simulink model "ctrl"  (R2018a)
settings: Solver=FixedStepDiscrete  StartTime=0.0  StopTime=3  RelTol=1e-3  EnableMultiTasking=on
undefined symbols (not defined in the file): AutoCalSt, Cfg_EnblLoadObs, Cfg_IndIDCntThshld, Cfg_IndIDCoolDownTicks, Cfg_IndIDMaxThshld, Cfg_IndIDMinThshld, Cfg_IndIDMtrVin, Cfg_IndIDSwTicks, Cfg_IndIDTs, Cfg_ResIDCntThshld, Cfg_ResIDMaxThshld, Cfg_ResIDMinThshld, Cfg_ResIDMtrVin, Cfg_SpdSnsSrc, DiscIntNeverNeededParam, MotorParams, MtrCtrlMd
libraries: ctrl_lib x5, simulink x3, adrc_lib x2
settings Model: PauseTimes=0.1  Creator=uids8840  LastModifiedBy=elrobotista
settings SolverCC: AutoInsertRateTranBlk=on
settings DataIOCC: SaveOutput=off  SignalLogging=off  DSMLogging=off  SaveTime=off
settings OptimizationCC: DefaultParameterBehavior=Inlined  UseFloatMulNetSlope=on  InlineInvariantSignals=on  PassReuseOutputArgsAs=Individual arguments  ZeroExternalMemoryAtStartup=off  ZeroInternalMemoryAtStartup=off  NoFixptDivByZeroProtection=on  EfficientFloat2IntCast=on  LifeSpan=1
settings DebuggingCC: ParameterTunabilityLossMsg=error
settings HardwareCC: ProdBitPerPointer=32  ProdBitPerSizeT=32  ProdBitPerPtrDiffT=32  ProdLargestAtomicInteger=Long  ProdLargestAtomicFloat=Double  ProdWordSize=32  ProdHWDeviceType=ARM Compatible->ARM Cortex
settings ModelReferenceCC: ModelReferenceNumInstancesAllowed=Single
settings SFSimCC: MATLABDynamicMemAlloc=off
settings RTWCC: SystemTargetFile=ert.tlc  GenCodeOnly=on  PackageGeneratedCodeAndArtifacts=on  PackageName=mtrctl  TemplateMakefile=ert_default_tmf  GenerateReport=on  IncludeHyperlinkInReport=on  LaunchReport=on  GenerateTraceInfo=on  GenerateTraceReport=on  GenerateTraceReportSl=on  GenerateTraceReportSf=on  GenerateTraceReportEml=on  GenerateCodeMetricsReport=on
settings CodeAppCC: ForceParamTrailComments=on  IgnoreCustomStorageClasses=off  OperatorAnnotations=on  SimulinkDataObjDesc=on  SFDataObjDesc=on  CustomSymbolStrGlobalVar=rt$N$M  CustomSymbolStrType=$N$M  CustomSymbolStrFcn=$N$M$F  CustomSymbolStrMacro=$N$M  InsertBlockDesc=on
settings ERTTargetCC: TargetLangStandard=C99 (ISO)  GenerateFullHeader=off  IncludeMdlTerminateFcn=off  CombineSignalStateStructs=on  SuppressErrorStatus=on  ERTCustomFileBanners=off  SupportAbsoluteTime=off  SupportNonFinite=off  SupportComplex=off  InlinedParameterPlacement=NonHierarchical  ERTCustomFileTemplate=example_file_process.tlc

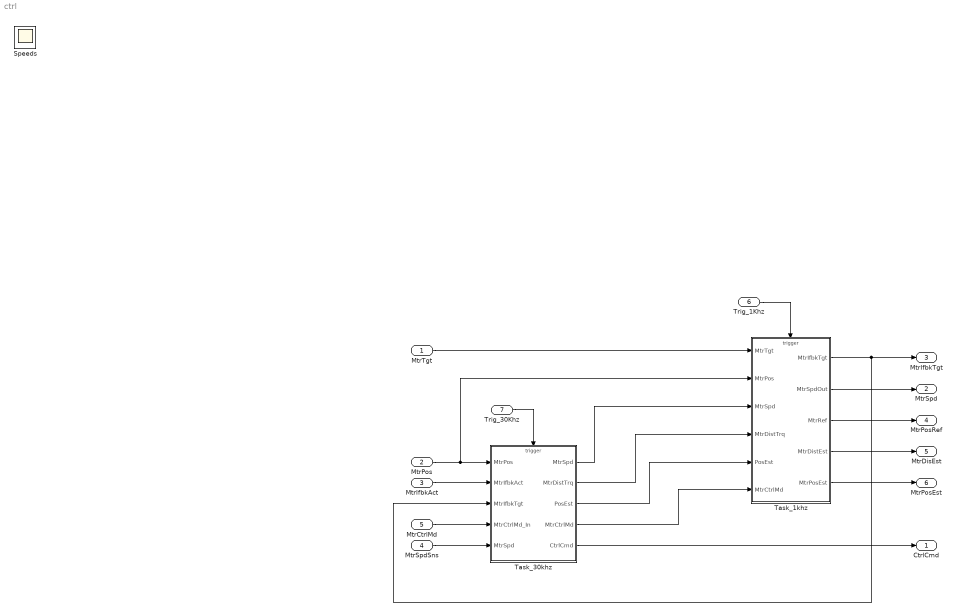
== system ctrl ==
  MtrTgt : Inport  OutDataTypeStr=single
  MtrPos : Inport  Port=2  OutDataTypeStr=single
  MtrIfbkAct : Inport  Port=3  OutDataTypeStr=single
  MtrSpdSns : Inport  Port=4
  MtrCtrlMd : Inport  Port=5  OutDataTypeStr=Enum: MtrCtrlMd
  Trig_1Khz : Inport  Port=6  OutputFunctionCall=on
  Trig_30Khz : Inport  Port=7  OutputFunctionCall=on
  Task_1khz : Subsystem  TreatAsAtomicUnit=on  SystemSampleTime=1/1e3
      settings: RTWFcnNameOpts=Use subsystem name  RTWFileNameOpts=Use function name  FunctionInterfaceSpec=Allow arguments
  Task_30khz : Subsystem  TreatAsAtomicUnit=on  SystemSampleTime=1/30e3
      settings: RTWFcnNameOpts=Use subsystem name  RTWFileNameOpts=Use subsystem name  FunctionInterfaceSpec=Allow arguments
  CtrlCmd : Outport
  MtrSpd : Outport  Port=2
  MtrIfbkTgt : Outport  Port=3
  MtrPosRef : Outport  Port=4
  MtrDisEst : Outport  Port=5
  MtrPosEst : Outport  Port=6
  Speeds : Scope
  wires:
  Task_30khz/1(MtrSpd) -> Task_1khz/3(MtrSpd)
  Trig_1Khz/1 -> Task_1khz/Trigger
  Trig_30Khz/1 -> Task_30khz/Trigger
  MtrIfbkAct/1 -> Task_30khz/2(MtrIfbkAct)
  MtrPos/1 -> Task_1khz/2(MtrPos), Task_30khz/1(" MtrPos")
  Task_1khz/2(MtrSpdOut) -> MtrSpd/1
  Task_1khz/1(MtrIfbkTgt) -> MtrIfbkTgt/1, Task_30khz/3(MtrIfbkTgt)
  MtrTgt/1 -> Task_1khz/1(MtrTgt)
  Task_1khz/3(MtrRef) -> MtrPosRef/1
  Task_1khz/4(MtrDistEst) -> MtrDisEst/1
  Task_1khz/5(MtrPosEst) -> MtrPosEst/1
  Task_30khz/5(CtrlCmd) -> CtrlCmd/1
  Task_30khz/2(MtrDistTrq) -> Task_1khz/4(MtrDistTrq)
  Task_30khz/3(PosEst) -> Task_1khz/5(PosEst)
  MtrCtrlMd/1 -> Task_30khz/4(MtrCtrlMd_In)
  MtrSpdSns/1 -> Task_30khz/5(" MtrSpd")
  Task_30khz/4(MtrCtrlMd) -> Task_1khz/6(MtrCtrlMd)

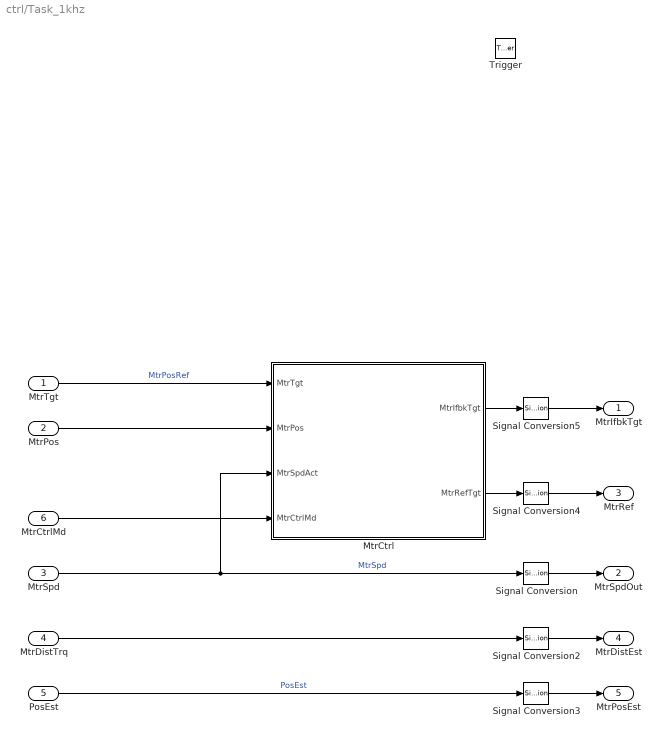
== system ctrl/Task_1khz ==
  MtrTgt : Inport
  MtrPos : Inport  Port=2
  MtrSpd : Inport  Port=3
  MtrDistTrq : Inport  Port=4
  PosEst : Inport  Port=5
  MtrCtrlMd : Inport  Port=6
  Trigger : TriggerPort  TriggerType=function-call  VariantControl=Variant  PortDimensions=1
  MtrCtrl : Subsystem
  Signal Conversion{,2..5} (5 alike) : SignalConversion  OverrideOpt=off
  MtrIfbkTgt : Outport
  MtrSpdOut : Outport  Port=2
  MtrRef : Outport  Port=3
  MtrDistEst : Outport  Port=4
  MtrPosEst : Outport  Port=5
  wires:
  MtrSpd/1 -> Signal Conversion/1, MtrCtrl/3(MtrSpdAct)  "MtrSpd"
  MtrCtrl/1(MtrIfbkTgt) -> Signal Conversion5/1
  Signal Conversion5/1 -> MtrIfbkTgt/1
  Signal Conversion/1 -> MtrSpdOut/1
  PosEst/1 -> Signal Conversion3/1  "PosEst"
  Signal Conversion2/1 -> MtrDistEst/1
  Signal Conversion3/1 -> MtrPosEst/1
  Signal Conversion4/1 -> MtrRef/1
  MtrTgt/1 -> MtrCtrl/1(MtrTgt)  "MtrPosRef"
  MtrCtrlMd/1 -> MtrCtrl/4(MtrCtrlMd)
  MtrDistTrq/1 -> Signal Conversion2/1
  MtrPos/1 -> MtrCtrl/2(MtrPos)
  MtrCtrl/2(MtrRefTgt) -> Signal Conversion4/1

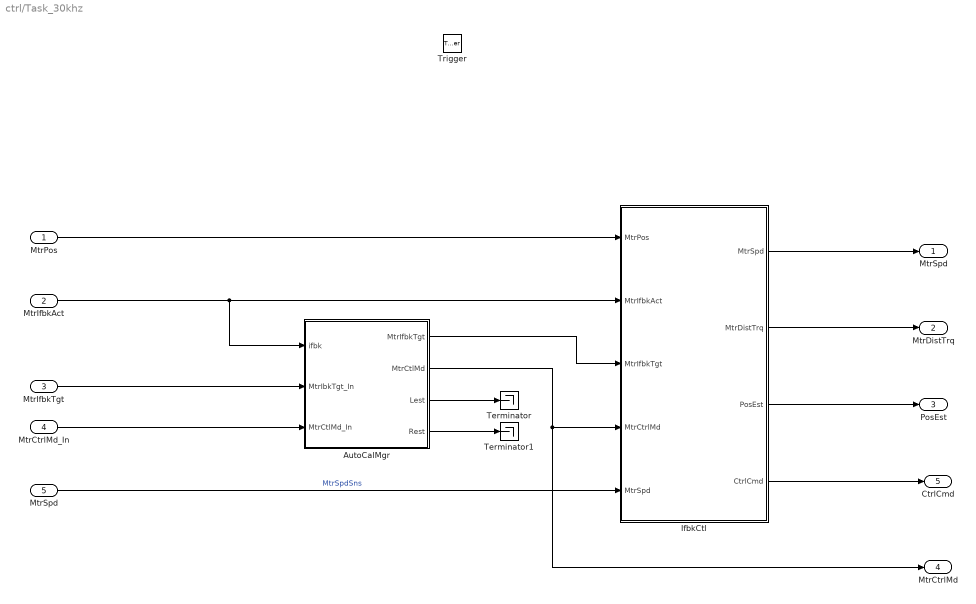
== system ctrl/Task_30khz ==
  " MtrPos" : Inport
  MtrIfbkAct : Inport  Port=2
  MtrIfbkTgt : Inport  Port=3
  MtrCtrlMd_In : Inport  Port=4
  " MtrSpd" : Inport  Port=5
  Trigger : TriggerPort  TriggerType=function-call  VariantControl=Variant  PortDimensions=1
  AutoCalMgr : Subsystem
  IfbkCtl : Subsystem
  Terminator : Terminator
  Terminator1 : Terminator
  MtrSpd : Outport
  MtrDistTrq : Outport  Port=2
  PosEst : Outport  Port=3
  MtrCtrlMd : Outport  Port=4
  CtrlCmd : Outport  Port=5
  wires:
  " MtrPos"/1 -> IfbkCtl/1(" MtrPos")
  " MtrSpd"/1 -> IfbkCtl/5(" MtrSpd")  "MtrSpdSns"
  IfbkCtl/1(MtrSpd) -> MtrSpd/1
  IfbkCtl/2(MtrDistTrq) -> MtrDistTrq/1
  IfbkCtl/3(PosEst) -> PosEst/1
  IfbkCtl/4(CtrlCmd) -> CtrlCmd/1
  MtrIfbkAct/1 -> IfbkCtl/2(MtrIfbkAct), AutoCalMgr/1(ifbk)
  AutoCalMgr/1(MtrIfbkTgt) -> IfbkCtl/3(MtrIfbkTgt)
  AutoCalMgr/3(Lest) -> Terminator/1
  AutoCalMgr/4(Rest) -> Terminator1/1
  MtrIfbkTgt/1 -> AutoCalMgr/2(MtrIbkTgt_In)
  MtrCtrlMd_In/1 -> AutoCalMgr/3(MtrCtlMd_In)
  AutoCalMgr/2(MtrCtlMd) -> MtrCtrlMd/1, IfbkCtl/4(MtrCtrlMd)

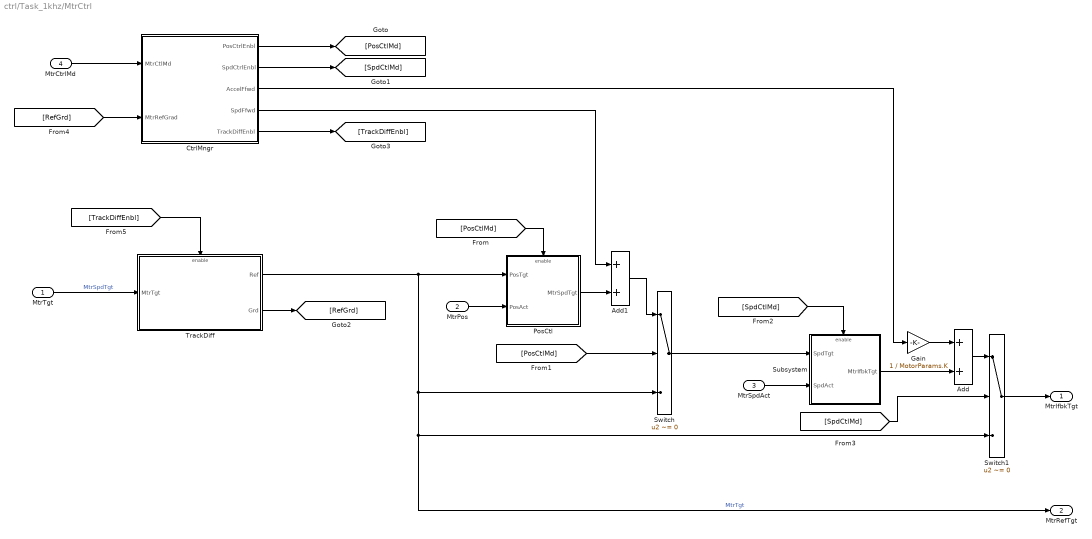
== system ctrl/Task_1khz/MtrCtrl ==
  MtrTgt : Inport
  MtrPos : Inport  Port=2
  MtrSpdAct : Inport  Port=3
  MtrCtrlMd : Inport  Port=4
  Add : Sum
  Add1 : Sum
  CtrlMngr : Subsystem
  Gain : Gain  Gain=1 / MotorParams.K
      settings: AttributesFormatString=%<Gain>
  PosCtl : Subsystem
  Subsystem : Subsystem
  Switch : Switch  Criteria=u2 ~= 0
  Switch1 : Switch  Criteria=u2 ~= 0
  TrackDiff : Subsystem  AncestorBlock=adrc_lib/TrackDiff  mask{ts=1e-3, h0=1e-3, r0=200}
      mask prompts: ts "Exeuction rate [s]:"
  MtrIfbkTgt : Outport
  MtrRefTgt : Outport  Port=2
  wires:
  MtrPos/1 -> PosCtl/2(PosAct)
  TrackDiff/1(Ref) -> PosCtl/1(PosTgt), Switch/3, Switch1/3, MtrRefTgt/1  "MtrTgt"
  [PosCtlMd] -> PosCtl/Enable
  [PosCtlMd] -> Switch/2
  Switch/1 -> Subsystem/1(SpdTgt)
  MtrSpdAct/1 -> Subsystem/2(SpdAct)
  [SpdCtlMd] -> Subsystem/Enable
  Switch1/1 -> MtrIfbkTgt/1
  [SpdCtlMd] -> Switch1/2
  Add/1 -> Switch1/1
  Subsystem/1(MtrIfbkTgt) -> Add/2
  PosCtl/1(MtrSpdTgt) -> Add1/2
  Add1/1 -> Switch/1
  MtrCtrlMd/1 -> CtrlMngr/1(MtrCtlMd)
  [RefGrd] -> CtrlMngr/2(MtrRefGrad)
  CtrlMngr/1(PosCtrlEnbl) -> [PosCtlMd]
  CtrlMngr/2(SpdCtrlEnbl) -> [SpdCtlMd]
  Gain/1 -> Add/1
  CtrlMngr/4(SpdFfwd) -> Add1/1
  CtrlMngr/3(AccelFfwd) -> Gain/1
  MtrTgt/1 -> TrackDiff/1(MtrTgt)  "MtrSpdTgt"
  TrackDiff/2(Grd) -> [RefGrd]
  CtrlMngr/5(TrackDiffEnbl) -> [TrackDiffEnbl]
  [TrackDiffEnbl] -> TrackDiff/Enable

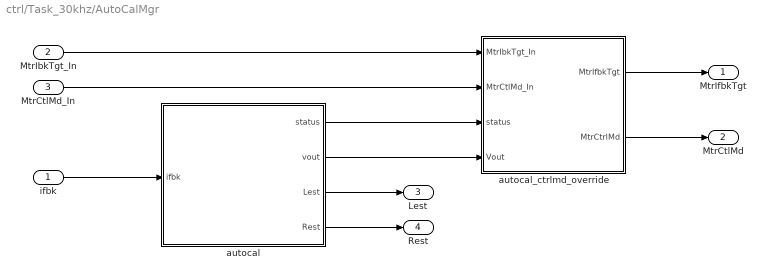
== system ctrl/Task_30khz/AutoCalMgr ==
  ifbk : Inport
  MtrIbkTgt_In : Inport  Port=2
  MtrCtlMd_In : Inport  Port=3
  autocal : Stateflow chart  TreatAsAtomicUnit=on
  autocal_ctrlmd_override : Subsystem
  MtrIfbkTgt : Outport
  MtrCtlMd : Outport  Port=2
  Lest : Outport  Port=3
  Rest : Outport  Port=4
  wires:
  ifbk/1 -> autocal/1(ifbk)
  autocal/3(Lest) -> Lest/1
  autocal/4(Rest) -> Rest/1
  MtrIbkTgt_In/1 -> autocal_ctrlmd_override/1(MtrIbkTgt_In)
  MtrCtlMd_In/1 -> autocal_ctrlmd_override/2(MtrCtlMd_In)
  autocal_ctrlmd_override/1(MtrIfbkTgt) -> MtrIfbkTgt/1
  autocal_ctrlmd_override/2(MtrCtrlMd) -> MtrCtlMd/1
  autocal/1(status) -> autocal_ctrlmd_override/3(status)
  autocal/2(vout) -> autocal_ctrlmd_override/4(Vout)

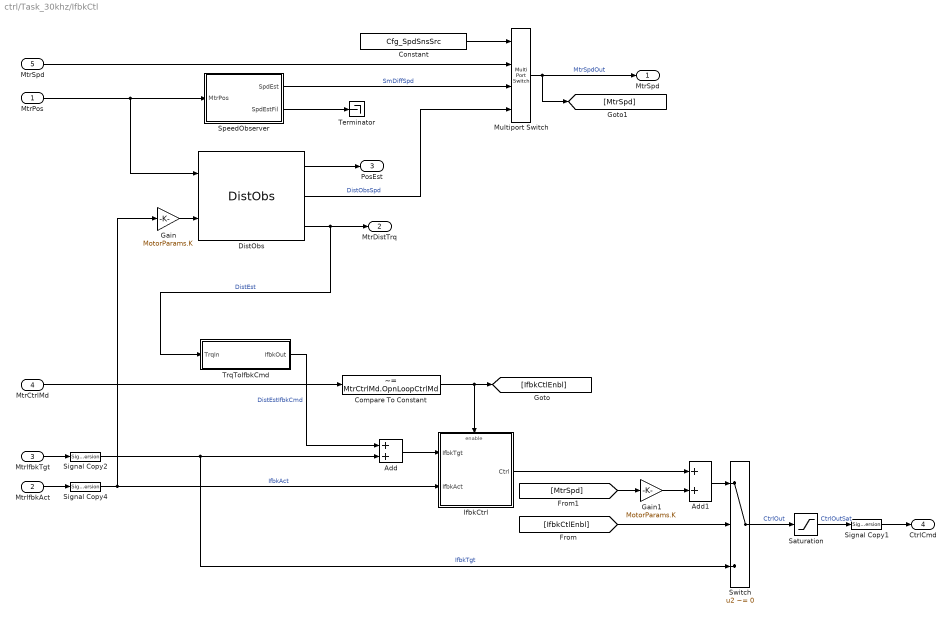
== system ctrl/Task_30khz/IfbkCtl ==
  " MtrPos" : Inport
  MtrIfbkAct : Inport  Port=2
  MtrIfbkTgt : Inport  Port=3
  MtrCtrlMd : Inport  Port=4
  " MtrSpd" : Inport  Port=5
  Add : Sum
  Add1 : Sum
  Compare To Constant : simulink/Logic and Bit Operations/Compare To Constant  relop=~=  const=MtrCtrlMd.OpnLoopCtrlMd  OutDataTypeStr=boolean
  Constant : Constant  Value=Cfg_SpdSnsSrc
  DistObs : adrc_lib/DistObs  ts=TsFast  Jm=DistObs_J  k1=DistObs_K1  k2=DistObs_K2  k3=DistObs_K3
  Gain : Gain  Gain=MotorParams.K
      settings: AttributesFormatString=%<Gain>
  Gain1 : Gain  Gain=MotorParams.K
      settings: AttributesFormatString=%<Gain>
  IfbkCtrl : Subsystem
  Multiport Switch : MultiPortSwitch  DataPortOrder=Zero-based contiguous  DiagnosticForDefault=None  zeroidx=on
  Saturation : Saturate  UpperLimit=12  LowerLimit=-12
  Signal Copy1 : SignalConversion  OverrideOpt=off
  Signal Copy2 : SignalConversion  OverrideOpt=off
  Signal Copy4 : SignalConversion  OverrideOpt=off
  SpeedObserver : Subsystem  RTWFcnName=SpdEst  RTWFileName=spdest
      settings: RTWFcnNameOpts=Use subsystem name  RTWFileNameOpts=Use subsystem name
  Switch : Switch  Criteria=u2 ~= 0
  Terminator : Terminator
  TrqToIfbkCmd : Subsystem
  MtrSpd : Outport
  MtrDistTrq : Outport  Port=2
  PosEst : Outport  Port=3
  CtrlCmd : Outport  Port=4
  wires:
  IfbkCtrl/1(Ctrl) -> Add1/1
  Add/1 -> IfbkCtrl/1(IfbkTgt)
  Compare To Constant/1 -> [IfbkCtlEnbl], IfbkCtrl/Enable
  DistObs/1 -> PosEst/1
  MtrIfbkTgt/1 -> Signal Copy2/1
  MtrCtrlMd/1 -> Compare To Constant/1
  Add1/1 -> Switch/1
  Signal Copy4/1 -> Gain/1, IfbkCtrl/2(IfbkAct)  "IfbkAct"
  Gain/1 -> DistObs/2
  Gain1/1 -> Add1/2
  Multiport Switch/1 -> MtrSpd/1, [MtrSpd]  "MtrSpdOut"
  Switch/1 -> Saturation/1  "CtrlOut"
  DistObs/2 -> Multiport Switch/4  "DistObsSpd"
  MtrIfbkAct/1 -> Signal Copy4/1
  " MtrSpd"/1 -> Multiport Switch/2
  Constant/1 -> Multiport Switch/1
  SpeedObserver/2(SpdEstFil) -> Terminator/1
  TrqToIfbkCmd/1(IfbkOut) -> Add/1  "DistEstIfbkCmd"
  [IfbkCtlEnbl] -> Switch/2
  Signal Copy2/1 -> Add/2, Switch/3  "IfbkTgt"
  SpeedObserver/1(SpdEst) -> Multiport Switch/3  "SmDiffSpd"
  " MtrPos"/1 -> DistObs/1, SpeedObserver/1(MtrPos)
  [MtrSpd] -> Gain1/1
  DistObs/3 -> MtrDistTrq/1, TrqToIfbkCmd/1(TrqIn)  "DistEst"
  Saturation/1 -> Signal Copy1/1  "CtrlOutSat"
  Signal Copy1/1 -> CtrlCmd/1

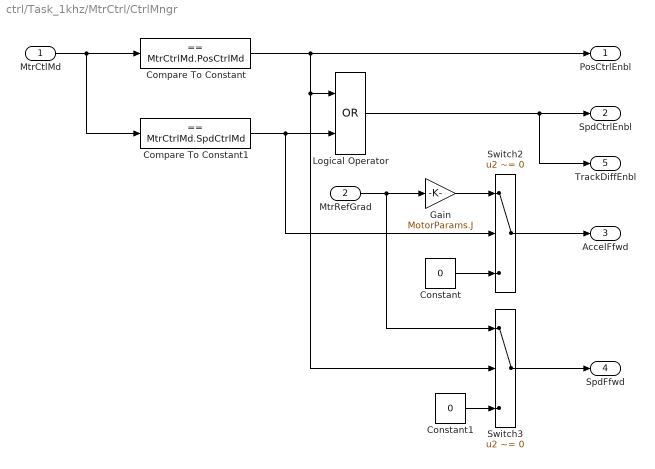
== system ctrl/Task_1khz/MtrCtrl/CtrlMngr ==
  MtrCtlMd : Inport
  MtrRefGrad : Inport  Port=2
  Compare To Constant : simulink/Logic and Bit Operations/Compare To Constant  relop===  const=MtrCtrlMd.PosCtrlMd  OutDataTypeStr=boolean
  Compare To Constant1 : simulink/Logic and Bit Operations/Compare To Constant  relop===  const=MtrCtrlMd.SpdCtrlMd  OutDataTypeStr=boolean
  Constant : Constant  Value=0  OutDataTypeStr=Inherit: Inherit via back propagation
  Constant1 : Constant  Value=0  OutDataTypeStr=Inherit: Inherit via back propagation
  Gain : Gain  Gain=MotorParams.J
      settings: AttributesFormatString=%<Gain>
  Logical Operator : Logic  Operator=OR  AllPortsSameDT=off  OutDataTypeStr=boolean
  Switch2 : Switch  Criteria=u2 ~= 0
  Switch3 : Switch  Criteria=u2 ~= 0
  PosCtrlEnbl : Outport
  SpdCtrlEnbl : Outport  Port=2
  AccelFfwd : Outport  Port=3
  SpdFfwd : Outport  Port=4
  TrackDiffEnbl : Outport  Port=5
  wires:
  Gain/1 -> Switch2/1
  Compare To Constant1/1 -> Logical Operator/2, Switch2/2
  Constant1/1 -> Switch3/3
  MtrRefGrad/1 -> Switch3/1, Gain/1
  Compare To Constant/1 -> PosCtrlEnbl/1, Switch3/2, Logical Operator/1
  Switch3/1 -> SpdFfwd/1
  Switch2/1 -> AccelFfwd/1
  Constant/1 -> Switch2/3
  MtrCtlMd/1 -> Compare To Constant1/1, Compare To Constant/1
  Logical Operator/1 -> TrackDiffEnbl/1, SpdCtrlEnbl/1

== system ctrl/Task_1khz/MtrCtrl/PosCtl ==
  PosTgt : Inport
  PosAct : Inport  Port=2
  Enable : EnablePort  StatesWhenEnabling=reset
  PI-Ctrl : ctrl_lib/PI-Ctrl  ts=TsMain  PI_Kp=PosCtrl_Kp  PI_Ki=0  max_lim=800  min_lim=-800
  MtrSpdTgt : Outport
  wires:
  PI-Ctrl/1 -> MtrSpdTgt/1  "MtrSpdTgt"
  PosTgt/1 -> PI-Ctrl/1
  PosAct/1 -> PI-Ctrl/2

== system ctrl/Task_1khz/MtrCtrl/Subsystem ==
  SpdTgt : Inport
  SpdAct : Inport  Port=2
  Enable : EnablePort  StatesWhenEnabling=reset
  PI-Ctrl1 : ctrl_lib/PI-Ctrl  ts=TsMain  PI_Kp=SpdCtrl_Kp  PI_Ki=SpdCtrl_Ki  max_lim=1.  min_lim=-1.
  MtrIfbkTgt : Outport
  wires:
  PI-Ctrl1/1 -> MtrIfbkTgt/1
  SpdAct/1 -> PI-Ctrl1/2
  SpdTgt/1 -> PI-Ctrl1/1

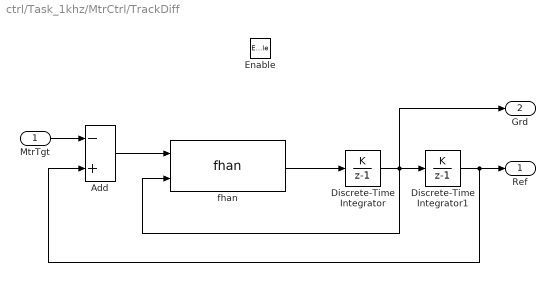
== system ctrl/Task_1khz/MtrCtrl/TrackDiff ==
  MtrTgt : Inport
  Enable : EnablePort  StatesWhenEnabling=reset
  Add : Sum  Inputs=-+
  Discrete-Time Integrator : DiscreteIntegrator  IntegratorMethod=Accumulation: Forward Euler  gainval=ts  SampleTime=-1  ICPrevOutput=DiscIntNeverNeededParam  ICPrevScaledInput=DiscIntNeverNeededParam
  Discrete-Time Integrator1 : DiscreteIntegrator  IntegratorMethod=Accumulation: Forward Euler  gainval=ts  SampleTime=-1  ICPrevOutput=DiscIntNeverNeededParam  ICPrevScaledInput=DiscIntNeverNeededParam
  fhan : adrc_lib/fhan  r0=r0  h0=h0
  Ref : Outport
  Grd : Outport  Port=2
  wires:
  MtrTgt/1 -> Add/1
  Add/1 -> fhan/1
  fhan/1 -> Discrete-Time Integrator/1
  Discrete-Time Integrator/1 -> Grd/1, fhan/2, Discrete-Time Integrator1/1
  Discrete-Time Integrator1/1 -> Add/2, Ref/1

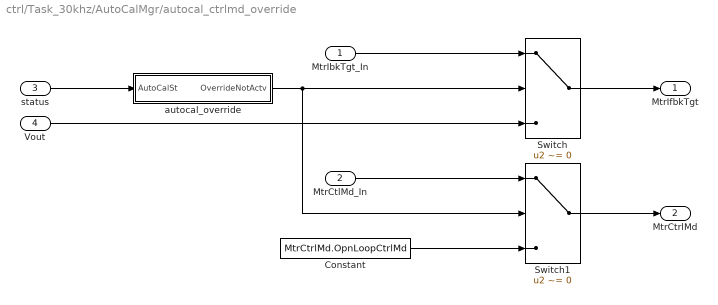
== system ctrl/Task_30khz/AutoCalMgr/autocal_ctrlmd_override ==
  MtrIbkTgt_In : Inport
  MtrCtlMd_In : Inport  Port=2
  status : Inport  Port=3
  Vout : Inport  Port=4
  Constant : Constant  Value=MtrCtrlMd.OpnLoopCtrlMd  OutDataTypeStr=Inherit: Inherit via back propagation
  Switch : Switch  Criteria=u2 ~= 0
  Switch1 : Switch  Criteria=u2 ~= 0
  autocal_override : Subsystem
  MtrIfbkTgt : Outport
  MtrCtrlMd : Outport  Port=2
  wires:
  Constant/1 -> Switch1/3
  MtrIbkTgt_In/1 -> Switch/1
  status/1 -> autocal_override/1(AutoCalSt)
  Vout/1 -> Switch/3
  autocal_override/1(OverrideNotActv) -> Switch/2, Switch1/2
  MtrCtlMd_In/1 -> Switch1/1
  Switch/1 -> MtrIfbkTgt/1
  Switch1/1 -> MtrCtrlMd/1

== system ctrl/Task_30khz/IfbkCtl/IfbkCtrl ==
  IfbkTgt : Inport
  IfbkAct : Inport  Port=2
  Enable : EnablePort  StatesWhenEnabling=reset
  IfbkCtrl : ctrl_lib/PI-Ctrl  ts=TsFast  PI_Kp=IfbkCtrl_Kp  PI_Ki=IfbkCtrl_Ki  max_lim=12  min_lim=-12.
  Ctrl : Outport
  wires:
  IfbkTgt/1 -> IfbkCtrl/1
  IfbkAct/1 -> IfbkCtrl/2
  IfbkCtrl/1 -> Ctrl/1

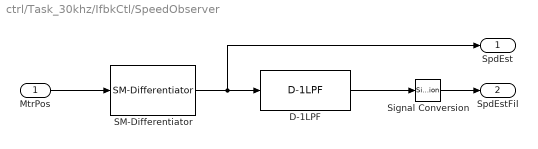
== system ctrl/Task_30khz/IfbkCtl/SpeedObserver ==
  MtrPos : Inport
  D-1LPF : ctrl_lib/D-1LPF  k_filt=SmDiff_FiltCnst
  SM-Differentiator : ctrl_lib/SM-Differentiator  sm_ki=SmDiff_Ki  sm_kp=SmDiff_Kp  ts=TsFast
  Signal Conversion : SignalConversion  OverrideOpt=off
  SpdEst : Outport
  SpdEstFil : Outport  Port=2
  wires:
  SM-Differentiator/1 -> SpdEst/1, D-1LPF/1
  D-1LPF/1 -> Signal Conversion/1
  MtrPos/1 -> SM-Differentiator/1
  Signal Conversion/1 -> SpdEstFil/1

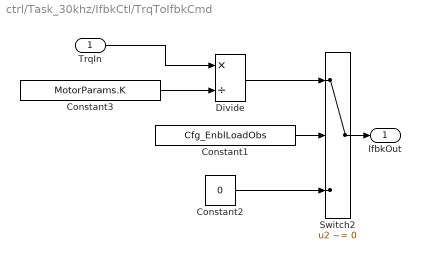
== system ctrl/Task_30khz/IfbkCtl/TrqToIfbkCmd ==
  TrqIn : Inport
  Constant1 : Constant  Value=Cfg_EnblLoadObs
  Constant2 : Constant  Value=0  OutDataTypeStr=Inherit: Inherit via back propagation
  Constant3 : Constant  Value=MotorParams.K  OutDataTypeStr=Inherit: Inherit via back propagation
  Divide : Product  Inputs=*/
  Switch2 : Switch  Criteria=u2 ~= 0
  IfbkOut : Outport
  wires:
  Constant2/1 -> Switch2/3
  Constant3/1 -> Divide/2
  Constant1/1 -> Switch2/2
  Divide/1 -> Switch2/1
  TrqIn/1 -> Divide/1
  Switch2/1 -> IfbkOut/1

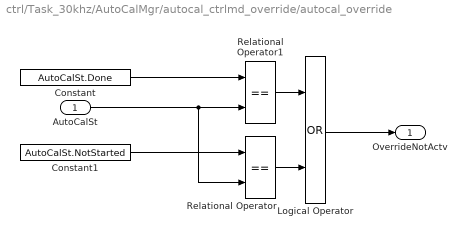
== system ctrl/Task_30khz/AutoCalMgr/autocal_ctrlmd_override/autocal_override ==
  AutoCalSt : Inport
  Constant : Constant  Value=AutoCalSt.Done  OutDataTypeStr=Inherit: Inherit via back propagation
  Constant1 : Constant  Value=AutoCalSt.NotStarted  OutDataTypeStr=Inherit: Inherit via back propagation
  Logical Operator : Logic  Operator=OR  AllPortsSameDT=off  OutDataTypeStr=boolean
  Relational Operator : RelationalOperator  Operator===  OutDataTypeStr=boolean  RndMeth=Simplest
  Relational Operator1 : RelationalOperator  Operator===  OutDataTypeStr=boolean  RndMeth=Simplest
  OverrideNotActv : Outport
  wires:
  Constant1/1 -> Relational Operator/1
  Constant/1 -> Relational Operator1/1
  Relational Operator/1 -> Logical Operator/2
  Relational Operator1/1 -> Logical Operator/1
  Logical Operator/1 -> OverrideNotActv/1
  AutoCalSt/1 -> Relational Operator/2, Relational Operator1/2

== stateflow chart ctrl/Task_30khz/AutoCalMgr/autocal ==
  state autocal_in_progress
    state inductance_id
      state inductance_switching
        entry:
        status = AutoCalSt.IndID;
        cycle_cnt = 0;
        state on_cycle
          entry:
          vout = Cfg_IndIDMtrVin;
          ifbk_neg += ifbk;
          cycle_cnt++;
        state off_cycle
          entry:
          vout = -Cfg_IndIDMtrVin;
          ifbk_pos += ifbk;
        (default) -> on_cycle
        on_cycle -> off_cycle : [after(Cfg_IndIDSwTicks, tick)]
        off_cycle -> on_cycle : [after(Cfg_IndIDSwTicks, tick)]
      state inductance_calc
        entry:
        Lest = Cfg_IndIDTs * Cfg_IndIDMtrVin * Cfg_IndIDCntThshld / (ifbk_pos - ifbk_neg);
        vout = Cfg_ResIDMtrVin;
        status = AutoCalSt.IndIDCoolDown;
      inductance_switching -> inductance_calc : [cycle_cnt >= Cfg_IndIDCntThshld]
    state resistance_id
      state resistance_id_on
        entry:
        status = AutoCalSt.ResID;
        ifbk_pos = 0;
        cycle_cnt = 0;
        vout = Cfg_ResIDMtrVin;
        during:
        ifbk_pos += ifbk;
        cycle_cnt++;
      state resistance_calc
        entry:
        Rest = Cfg_ResIDMtrVin * Cfg_ResIDCntThshld / ifbk_pos;
        vout = 0;
      resistance_id_on -> resistance_calc : [cycle_cnt >= Cfg_ResIDCntThshld]
    inductance_calc -> resistance_id_on [order 2] : [after(Cfg_IndIDCoolDownTicks, tick)]
  state autocal_resistance_error
    entry:
    vout = 0;
    state resistance_too_small
      entry:
      status = AutoCalSt.ErrResTooSmall;
    state resistance_too_large
      entry:
      status = AutoCalSt.ErrResTooLarge;
  state autocal_inductance_error
    entry:
    vout = 0;
    state inductance_too_large
      entry:
      status = AutoCalSt.ErrIndTooLarge;
    state inductance_too_small
      entry:
      status = AutoCalSt.ErrIndTooSmall;
  state autocal_done
    entry:
    status = AutoCalSt.Done;
    vout = 0;
  (default) -> inductance_switching
  resistance_calc -> resistance_too_small [order 1] : [Rest <= Cfg_ResIDMinThshld]
  resistance_calc -> resistance_too_large [order 2] : [Rest >= Cfg_ResIDMaxThshld]
  inductance_calc -> inductance_too_large [order 1] : [Lest >= Cfg_IndIDMaxThshld]
  resistance_calc -> autocal_done [order 3]
  inductance_calc -> inductance_too_small [order 3] : [Lest <= Cfg_IndIDMinThshld]
  data: status output Enum: AutoCalSt size=1 =AutoCalSt.NotStarted; cycle_cnt local int32 size=1 =0; ifbk input single size=1; vout output single size=1 =0; ifbk_neg local single size=1 =0; ifbk_pos local single size=1 =0; Cfg_IndIDCntThshld parameter; Lest output single size=1 =-1; Cfg_ResIDCntThshld parameter; Rest output single size=1 =-1; Cfg_IndIDMtrVin parameter; Cfg_IndIDCoolDownTicks parameter; Cfg_IndIDSwTicks parameter; Cfg_IndIDTs parameter; Cfg_ResIDMtrVin parameter; Cfg_IndIDMaxThshld parameter; Cfg_IndIDMinThshld parameter; Cfg_ResIDMinThshld parameter; Cfg_ResIDMaxThshld parameter
